simulink model "S_Fun_GetSet"  (R2020b)
settings: Solver=VariableStepAuto  StartTime=0.0  StopTime=10.0  RelTol=1e-3
undefined symbols (not defined in the file): object
settings Model: Creator=yinti  LastModifiedBy=yinti

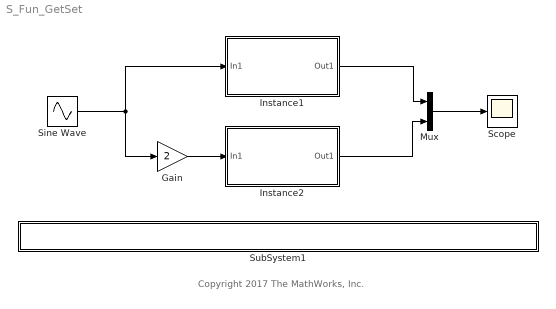
== system S_Fun_GetSet ==
  note: Copyright 2017 The MathWorks, Inc.
  Gain : Gain  Gain=2
  Instance1 : Subsystem
  Instance2 : Subsystem
  Mux : Mux  Inputs=2
  Scope : Scope
  Sine Wave : Sin  Phase=pi/2  SampleTime=0
  SubSystem1 : Subsystem  mask{filename=sfun_simulinkfunction_getset.cpp}
      mask init:
      | x=sfundemo_maskdisp;
      settings: AttributesFormatString=\n  OpenFcn=sfundemo_openfcn
      mask Display: disp(x);
  wires:
  Instance2/1(Out1) -> Mux/2
  Sine Wave/1 -> Gain/1, Instance1/1(In1)
  Instance1/1(Out1) -> Mux/1
  Gain/1 -> Instance2/1(In1)
  Mux/1 -> Scope/1

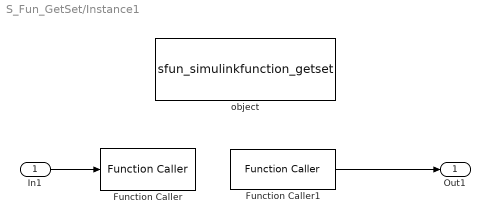
== system S_Fun_GetSet/Instance1 ==
  In1 : Inport
  Function Caller : FunctionCaller  Priority=1  FunctionPrototype=object.set(u)  InputArgumentSpecifications=<Enter example>  OutputArgumentSpecifications=<Enter example>
  Function Caller1 : FunctionCaller  Priority=2  FunctionPrototype=y = object.get()  InputArgumentSpecifications=<Enter example>  OutputArgumentSpecifications=<Enter example>
  object : S-Function  FunctionName=sfun_simulinkfunction_getset  SFunctionDeploymentMode=off  EnableBusSupport=off
  Out1 : Outport  VectorParamsAs1DForOutWhenUnconnected=off
  wires:
  In1/1 -> Function Caller/1
  Function Caller1/1 -> Out1/1

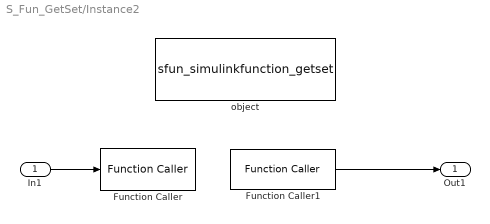
== system S_Fun_GetSet/Instance2 ==
  In1 : Inport
  Function Caller : FunctionCaller  Priority=1  FunctionPrototype=object.set(u)  InputArgumentSpecifications=<Enter example>  OutputArgumentSpecifications=<Enter example>
  Function Caller1 : FunctionCaller  Priority=2  FunctionPrototype=y = object.get()  InputArgumentSpecifications=<Enter example>  OutputArgumentSpecifications=<Enter example>
  object : S-Function  FunctionName=sfun_simulinkfunction_getset  SFunctionDeploymentMode=off  EnableBusSupport=off
  Out1 : Outport  VectorParamsAs1DForOutWhenUnconnected=off
  wires:
  Function Caller1/1 -> Out1/1
  In1/1 -> Function Caller/1

== system S_Fun_GetSet/SubSystem1 ==
